simulink model "proxy"  (R2017b)
settings: Solver=ode3  StartTime=0.0  StopTime=inf  FixedStep=0.01  RelTol=1e-3  EnableMultiTasking=on
model workspace (MAT data in the model file):
  SL_ROS_VariableLengthArrays_MaxSizes : struct (value not decoded)
values from neighbouring files (symbols this model uses):
  filt = c2d(filt,sampleTime)    [Connect.m]
libraries: robotlib x8, simulink x6, simulink_extras x3, dspnetwork x3, etargetslib x2, xpcutilitieslib x1
(part 3 of 4)

== matlab function proxy/Generate SchunkCommands /Middle Finger/Jacobian2 ==
  data: pose input; sensor input; measurements input; JTcomp output single; q_next output; q_pr input; J22_old input; J22_ol output
function [JTcomp, q_next, J22_ol] = fcn( pose, sensor, measurements, q_pr, J22_old)
%#codegen
% JTcomp_T = zeros(1,2);
%JTcomp = zeros(1,2);

lx = sensor(1);
qB = sensor(2);

qo1 =pose(1);
qo2 =pose(2);
qK = pose(3);
qD = pose(4);
qG = pose(5);
qN = pose(6);
c1 = pose(7);
c2 = pose(8);

%POSE ESTIMATION VALUE
LIIp = measurements(2);
LJJp = LIIp;
LLM = measurements(1);

%LIIp= measurements(1);
%LJJp = measurements(2);
%LLM = measurements(3);
%offset = measurements(4);
%xL = measurements(5);


% LIIp = 7;
% LJJp = LIIp;
% LLM = 50;
% offset = 3;
xL = 10;

f1 = LLM;
f5 = xL;
LBH = 37; 
LKB = 35;
LKH = LKB + LBH;
LCI = 16;
LGH =  86;
LHG =  LGH;
LDE = 40;
LAB =  18;   
LEF =  27;
LGF =  46;
LCD =  9;
LBC =  43;
oy  = 134.8;
ox  = 15; 
LEJ =  39;
off_fing = LIIp;  
lact = 117.77;
% LKN =  135.6320;
LNO = lact;
LDF = LDE + LEF;
LBD = LBC + LCD;


stepsize = 0.01;

%%NEWEST (Jacobian_StiffnessRenderingOptimization_Sim.mdl)
q_dif = (sensor - q_pr) / stepsize;
q_dif1 = q_dif(1);
q_dif2 = q_dif(2);


J11 = -(cos(qo1)*(LKB*cos(qK)+LBC*cos(qB-qK)-LCI*sin(qB-qK))-sin(qo1)*(LKB*sin(qK)-LBC*sin(qB-qK)-LCI*cos(qB-qK)))*((LDE+LEF)*sin(qo2)*cos(qB-qD-qG)*(LKB*sin(qK)-LBC*sin(qB-qK)-LCI*cos(qB-qK))+(LDE+LEF)*sin(qN)^2*cos(qB-qD-qG)*(cos(qo1)*sin(qo1+qo2)*(LKB*sin(qK)-LBC*sin(qB-qK))-LCI*cos(qo1)*sin(qo1+qo2)*cos(qB-qK)-sin(qo2)*(LKB*sin(qK)-LBC*sin(qB-qK)-LCI*cos(qB-qK))-sin(qo1)*cos(qo1+qo2)*(LKB*sin(qK)-LBC*sin(qB-qK)-LCI*cos(qB-qK)))-cos(qo1)*((LDE+LEF)*cos(qB-qD-qG)*(cos(qo1+qo2)*(LCD*cos(qB-qK)+LCI*sin(qB-qK)+LDE*cos(qB-qD-qK)-LEJ*sin(qB-qD-qK))-sin(qo1+qo2)*(LCI*cos(qB-qK)-LCD*sin(qB-qK)-LDE*sin(qB-qD-qK)-LEJ*cos(qB-qD-qK)))+(sin(qo1+qo2)*(LDE*sin(qB-qD-qK)+LEJ*cos(qB-qD-qK))+cos(qo1+qo2)*(LDE*cos(qB-qD-qK)-LEJ*sin(qB-qD-qK)))*(cos(qG-qK)*(LBH*cos(qK)+LHG*sin(qK)-LBC*cos(qB-qK)-LCD*cos(qB-qK)-LDE*cos(qB-qD-qK)-LEF*cos(qB-qD-qK))+sin(qG-qK)*(LHG*cos(qK)-LBH*sin(qK)-LBC*sin(qB-qK)-LCD*sin(qB-qK)-LDE*sin(qB-qD-qK)-LEF*sin(qB-qD-qK)))))/(cos(qN)*(LKB*sin(qK)+LAB*sin(qB-qK)-tan(qN)*(LKB*cos(qK)-LAB*cos(qB-qK)))*((LDE+LEF)*sin(qo1)*sin(qo2)*cos(qB-qD-qG)*(LIIp*cos(qo1)-c1*sin(qo1))*(LKB*sin(qK)-LBC*sin(qB-qK)-LCI*cos(qB-qK))-cos(qo1)*((LIIp*sin(qo1)+c1*cos(qo1))*((LDE+LEF)*sin(qo2)*cos(qB-qD-qG)*(LKB*sin(qK)-LBC*sin(qB-qK)-LCI*cos(qB-qK))-cos(qo1)*((LDE+LEF)*cos(qB-qD-qG)*(cos(qo1+qo2)*(LCD*cos(qB-qK)+LCI*sin(qB-qK)+LDE*cos(qB-qD-qK)-LEJ*sin(qB-qD-qK))-sin(qo1+qo2)*(LCI*cos(qB-qK)-LCD*sin(qB-qK)-LDE*sin(qB-qD-qK)-LEJ*cos(qB-qD-qK)))+(sin(qo1+qo2)*(LDE*sin(qB-qD-qK)+LEJ*cos(qB-qD-qK))+cos(qo1+qo2)*(LDE*cos(qB-qD-qK)-LEJ*sin(qB-qD-qK)))*(cos(qG-qK)*(LBH*cos(qK)+LHG*sin(qK)-LBC*cos(qB-qK)-LCD*cos(qB-qK)-LDE*cos(qB-qD-qK)-LEF*cos(qB-qD-qK))+sin(qG-qK)*(LHG*cos(qK)-LBH*sin(qK)-LBC*sin(qB-qK)-LCD*sin(qB-qK)-LDE*sin(qB-qD-qK)-LEF*sin(qB-qD-qK)))))-sin(qo1)*(LIIp*cos(qo1)-c1*sin(qo1))*((LDE+LEF)*sin(qo1+qo2)*cos(qB-qD-qG)*(LCI*cos(qB-qK)-LCD*sin(qB-qK)-LDE*sin(qB-qD-qK)-LEJ*cos(qB-qD-qK))-sin(qo1+qo2)*(LDE*sin(qB-qD-qK)+LEJ*cos(qB-qD-qK))*(cos(qG-qK)*(LBH*cos(qK)+LHG*sin(qK)-LBC*cos(qB-qK)-LCD*cos(qB-qK)-LDE*cos(qB-qD-qK)-LEF*cos(qB-qD-qK))+sin(qG-qK)*(LHG*cos(qK)-LBH*sin(qK)-LBC*sin(qB-qK)-LCD*sin(qB-qK)-LDE*sin(qB-qD-qK)-LEF*sin(qB-qD-qK)))-cos(qo1+qo2)*((LDE+LEF)*cos(qG-qK)*cos(qB-qD-qK)*(LCD*cos(qB-qK)+LCI*sin(qB-qK)+LDE*cos(qB-qD-qK)-LEJ*sin(qB-qD-qK))+cos(qG-qK)*(LDE*cos(qB-qD-qK)-LEJ*sin(qB-qD-qK))*(LBH*cos(qK)+LHG*sin(qK)-LBC*cos(qB-qK)-LCD*cos(qB-qK)-LDE*cos(qB-qD-qK)-LEF*cos(qB-qD-qK))+sin(qG-qK)*((LDE+LEF)*sin(qB-qD-qK)*(LCD*cos(qB-qK)+LCI*sin(qB-qK)+LDE*cos(qB-qD-qK)-LEJ*sin(qB-qD-qK))+(LDE*cos(qB-qD-qK)-LEJ*sin(qB-qD-qK))*(LHG*cos(qK)-LBH*sin(qK)-LBC*sin(qB-qK)-LCD*sin(qB-qK)-LDE*sin(qB-qD-qK)-LEF*sin(qB-qD-qK))))))));
J12 = cos(qo1)*((LDE+LEF)*sin(qo1+qo2)*cos(qB-qD-qG)*(LCI*cos(qB-qK)-LCD*sin(qB-qK)-LDE*sin(qB-qD-qK)-LEJ*cos(qB-qD-qK))*(cos(qo1)*(LKB*cos(qK)+LBC*cos(qB-qK)-LCI*sin(qB-qK))-sin(qo1)*(LKB*sin(qK)-LBC*sin(qB-qK)-LCI*cos(qB-qK)))+sin(qG-qK)*(LBC*sin(qB-qK)+LCD*sin(qB-qK)+LDE*sin(qB-qD-qK)+LEF*sin(qB-qD-qK))*(sin(qo1+qo2)*(LDE*sin(qB-qD-qK)+LEJ*cos(qB-qD-qK))+cos(qo1+qo2)*(LDE*cos(qB-qD-qK)-LEJ*sin(qB-qD-qK)))*(cos(qo1)*(LKB*cos(qK)+LBC*cos(qB-qK)-LCI*sin(qB-qK))-sin(qo1)*(LKB*sin(qK)-LBC*sin(qB-qK)-LCI*cos(qB-qK)))+cos(qG-qK)*(LBC*cos(qB-qK)+LCD*cos(qB-qK)+LDE*cos(qB-qD-qK)+LEF*cos(qB-qD-qK))*(sin(qo1+qo2)*(LDE*sin(qB-qD-qK)+LEJ*cos(qB-qD-qK))+cos(qo1+qo2)*(LDE*cos(qB-qD-qK)-LEJ*sin(qB-qD-qK)))*(cos(qo1)*(LKB*cos(qK)+LBC*cos(qB-qK)-LCI*sin(qB-qK))-sin(qo1)*(LKB*sin(qK)-LBC*sin(qB-qK)-LCI*cos(qB-qK)))-(LDE+LEF)*cos(qo1+qo2)*cos(qB-qD-qG)*(LCD*cos(qB-qK)+LCI*sin(qB-qK)+LDE*cos(qB-qD-qK)-LEJ*sin(qB-qD-qK))*(cos(qo1)*(LKB*cos(qK)+LBC*cos(qB-qK)-LCI*sin(qB-qK))-sin(qo1)*(LKB*sin(qK)-LBC*sin(qB-qK)-LCI*cos(qB-qK)))-(LBC*cos(qB-qK)-LCI*sin(qB-qK))*((LDE+LEF)*sin(qo2)*cos(qB-qD-qG)*(LKB*sin(qK)-LBC*sin(qB-qK)-LCI*cos(qB-qK))-cos(qo1)*((LDE+LEF)*cos(qB-qD-qG)*(cos(qo1+qo2)*(LCD*cos(qB-qK)+LCI*sin(qB-qK)+LDE*cos(qB-qD-qK)-LEJ*sin(qB-qD-qK))-sin(qo1+qo2)*(LCI*cos(qB-qK)-LCD*sin(qB-qK)-LDE*sin(qB-qD-qK)-LEJ*cos(qB-qD-qK)))+(sin(qo1+qo2)*(LDE*sin(qB-qD-qK)+LEJ*cos(qB-qD-qK))+cos(qo1+qo2)*(LDE*cos(qB-qD-qK)-LEJ*sin(qB-qD-qK)))*(cos(qG-qK)*(LBH*cos(qK)+LHG*sin(qK)-LBC*cos(qB-qK)-LCD*cos(qB-qK)-LDE*cos(qB-qD-qK)-LEF*cos(qB-qD-qK))+sin(qG-qK)*(LHG*cos(qK)-LBH*sin(qK)-LBC*sin(qB-qK)-LCD*sin(qB-qK)-LDE*sin(qB-qD-qK)-LEF*sin(qB-qD-qK)))))-(LBC*sin(qB-qK)+LCI*cos(qB-qK))*((LDE+LEF)*sin(qo2)*cos(qB-qD-qG)*(LKB*cos(qK)+LBC*cos(qB-qK)-LCI*sin(qB-qK))+sin(qo1)*((LDE+LEF)*sin(qo1+qo2)*cos(qB-qD-qG)*(LCI*cos(qB-qK)-LCD*sin(qB-qK)-LDE*sin(qB-qD-qK)-LEJ*cos(qB-qD-qK))-sin(qo1+qo2)*(LDE*sin(qB-qD-qK)+LEJ*cos(qB-qD-qK))*(cos(qG-qK)*(LBH*cos(qK)+LHG*sin(qK)-LBC*cos(qB-qK)-LCD*cos(qB-qK)-LDE*cos(qB-qD-qK)-LEF*cos(qB-qD-qK))+sin(qG-qK)*(LHG*cos(qK)-LBH*sin(qK)-LBC*sin(qB-qK)-LCD*sin(qB-qK)-LDE*sin(qB-qD-qK)-LEF*sin(qB-qD-qK)))-cos(qo1+qo2)*((LDE+LEF)*cos(qG-qK)*cos(qB-qD-qK)*(LCD*cos(qB-qK)+LCI*sin(qB-qK)+LDE*cos(qB-qD-qK)-LEJ*sin(qB-qD-qK))+cos(qG-qK)*(LDE*cos(qB-qD-qK)-LEJ*sin(qB-qD-qK))*(LBH*cos(qK)+LHG*sin(qK)-LBC*cos(qB-qK)-LCD*cos(qB-qK)-LDE*cos(qB-qD-qK)-LEF*cos(qB-qD-qK))+sin(qG-qK)*((LDE+LEF)*sin(qB-qD-qK)*(LCD*cos(qB-qK)+LCI*sin(qB-qK)+LDE*cos(qB-qD-qK)-LEJ*sin(qB-qD-qK))+(LDE*cos(qB-qD-qK)-LEJ*sin(qB-qD-qK))*(LHG*cos(qK)-LBH*sin(qK)-LBC*sin(qB-qK)-LCD*sin(qB-qK)-LDE*sin(qB-qD-qK)-LEF*sin(qB-qD-qK)))))))/((LDE+LEF)*sin(qo1)*sin(qo2)*cos(qB-qD-qG)*(LIIp*cos(qo1)-c1*sin(qo1))*(LKB*sin(qK)-LBC*sin(qB-qK)-LCI*cos(qB-qK))-cos(qo1)*((LIIp*sin(qo1)+c1*cos(qo1))*((LDE+LEF)*sin(qo2)*cos(qB-qD-qG)*(LKB*sin(qK)-LBC*sin(qB-qK)-LCI*cos(qB-qK))-cos(qo1)*((LDE+LEF)*cos(qB-qD-qG)*(cos(qo1+qo2)*(LCD*cos(qB-qK)+LCI*sin(qB-qK)+LDE*cos(qB-qD-qK)-LEJ*sin(qB-qD-qK))-sin(qo1+qo2)*(LCI*cos(qB-qK)-LCD*sin(qB-qK)-LDE*sin(qB-qD-qK)-LEJ*cos(qB-qD-qK)))+(sin(qo1+qo2)*(LDE*sin(qB-qD-qK)+LEJ*cos(qB-qD-qK))+cos(qo1+qo2)*(LDE*cos(qB-qD-qK)-LEJ*sin(qB-qD-qK)))*(cos(qG-qK)*(LBH*cos(qK)+LHG*sin(qK)-LBC*cos(qB-qK)-LCD*cos(qB-qK)-LDE*cos(qB-qD-qK)-LEF*cos(qB-qD-qK))+sin(qG-qK)*(LHG*cos(qK)-LBH*sin(qK)-LBC*sin(qB-qK)-LCD*sin(qB-qK)-LDE*sin(qB-qD-qK)-LEF*sin(qB-qD-qK)))))-sin(qo1)*(LIIp*cos(qo1)-c1*sin(qo1))*((LDE+LEF)*sin(qo1+qo2)*cos(qB-qD-qG)*(LCI*cos(qB-qK)-LCD*sin(qB-qK)-LDE*sin(qB-qD-qK)-LEJ*cos(qB-qD-qK))-sin(qo1+qo2)*(LDE*sin(qB-qD-qK)+LEJ*cos(qB-qD-qK))*(cos(qG-qK)*(LBH*cos(qK)+LHG*sin(qK)-LBC*cos(qB-qK)-LCD*cos(qB-qK)-LDE*cos(qB-qD-qK)-LEF*cos(qB-qD-qK))+sin(qG-qK)*(LHG*cos(qK)-LBH*sin(qK)-LBC*sin(qB-qK)-LCD*sin(qB-qK)-LDE*sin(qB-qD-qK)-LEF*sin(qB-qD-qK)))-cos(qo1+qo2)*((LDE+LEF)*cos(qG-qK)*cos(qB-qD-qK)*(LCD*cos(qB-qK)+LCI*sin(qB-qK)+LDE*cos(qB-qD-qK)-LEJ*sin(qB-qD-qK))+cos(qG-qK)*(LDE*cos(qB-qD-qK)-LEJ*sin(qB-qD-qK))*(LBH*cos(qK)+LHG*sin(qK)-LBC*cos(qB-qK)-LCD*cos(qB-qK)-LDE*cos(qB-qD-qK)-LEF*cos(qB-qD-qK))+sin(qG-qK)*((LDE+LEF)*sin(qB-qD-qK)*(LCD*cos(qB-qK)+LCI*sin(qB-qK)+LDE*cos(qB-qD-qK)-LEJ*sin(qB-qD-qK))+(LDE*cos(qB-qD-qK)-LEJ*sin(qB-qD-qK))*(LHG*cos(qK)-LBH*sin(qK)-LBC*sin(qB-qK)-LCD*sin(qB-qK)-LDE*sin(qB-qD-qK)-LEF*sin(qB-qD-qK))))))) - (cos(qo1)*(LKB*cos(qK)+LBC*cos(qB-qK)-LCI*sin(qB-qK))-sin(qo1)*(LKB*sin(qK)-LBC*sin(qB-qK)-LCI*cos(qB-qK)))*((LDE+LEF)*cos(qo1)*sin(qo1+qo2)*cos(qB-qD-qG)*(LKB*sin(qK)+LAB*sin(qB-qK)-tan(qN)*(LKB*cos(qK)-LAB*cos(qB-qK)))*(LCI*cos(qB-qK)-LCD*sin(qB-qK)-LDE*sin(qB-qD-qK)-LEJ*cos(qB-qD-qK))+cos(qo1)*sin(qG-qK)*(LKB*sin(qK)+LAB*sin(qB-qK)-tan(qN)*(LKB*cos(qK)-LAB*cos(qB-qK)))*(LBC*sin(qB-qK)+LCD*sin(qB-qK)+LDE*sin(qB-qD-qK)+LEF*sin(qB-qD-qK))*(sin(qo1+qo2)*(LDE*sin(qB-qD-qK)+LEJ*cos(qB-qD-qK))+cos(qo1+qo2)*(LDE*cos(qB-qD-qK)-LEJ*sin(qB-qD-qK)))+cos(qo1)*cos(qG-qK)*(LKB*sin(qK)+LAB*sin(qB-qK)-tan(qN)*(LKB*cos(qK)-LAB*cos(qB-qK)))*(LBC*cos(qB-qK)+LCD*cos(qB-qK)+LDE*cos(qB-qD-qK)+LEF*cos(qB-qD-qK))*(sin(qo1+qo2)*(LDE*sin(qB-qD-qK)+LEJ*cos(qB-qD-qK))+cos(qo1+qo2)*(LDE*cos(qB-qD-qK)-LEJ*sin(qB-qD-qK)))-(LDE+LEF)*sin(qo2)*cos(qB-qD-qG)*(LBC*sin(qB-qK)+LCI*cos(qB-qK))*(LKB*sin(qK)+LAB*sin(qB-qK)-tan(qN)*(LKB*cos(qK)-LAB*cos(qB-qK)))-(LDE+LEF)*cos(qo1)*cos(qo1+qo2)*cos(qB-qD-qG)*(LKB*sin(qK)+LAB*sin(qB-qK)-tan(qN)*(LKB*cos(qK)-LAB*cos(qB-qK)))*(LCD*cos(qB-qK)+LCI*sin(qB-qK)+LDE*cos(qB-qD-qK)-LEJ*sin(qB-qD-qK))-LAB*sin(qB-qK)*((LDE+LEF)*sin(qo2)*cos(qB-qD-qG)*(LKB*sin(qK)-LBC*sin(qB-qK)-LCI*cos(qB-qK))-cos(qo1)*((LDE+LEF)*cos(qB-qD-qG)*(cos(qo1+qo2)*(LCD*cos(qB-qK)+LCI*sin(qB-qK)+LDE*cos(qB-qD-qK)-LEJ*sin(qB-qD-qK))-sin(qo1+qo2)*(LCI*cos(qB-qK)-LCD*sin(qB-qK)-LDE*sin(qB-qD-qK)-LEJ*cos(qB-qD-qK)))+(sin(qo1+qo2)*(LDE*sin(qB-qD-qK)+LEJ*cos(qB-qD-qK))+cos(qo1+qo2)*(LDE*cos(qB-qD-qK)-LEJ*sin(qB-qD-qK)))*(cos(qG-qK)*(LBH*cos(qK)+LHG*sin(qK)-LBC*cos(qB-qK)-LCD*cos(qB-qK)-LDE*cos(qB-qD-qK)-LEF*cos(qB-qD-qK))+sin(qG-qK)*(LHG*cos(qK)-LBH*sin(qK)-LBC*sin(qB-qK)-LCD*sin(qB-qK)-LDE*sin(qB-qD-qK)-LEF*sin(qB-qD-qK)))))-LAB*tan(qN)*cos(qB-qK)*((LDE+LEF)*cos(qo1)*sin(qo1+qo2)*cos(qB-qD-qG)*(LKB*sin(qK)-LBC*sin(qB-qK)-LCD*sin(qB-qK)-LDE*sin(qB-qD-qK)-LEJ*cos(qB-qD-qK))-(LDE+LEF)*sin(qo1)*cos(qo1+qo2)*cos(qB-qD-qG)*(LKB*sin(qK)-LBC*sin(qB-qK)-LCI*cos(qB-qK))-cos(qo1)*sin(qo1+qo2)*(LDE*sin(qB-qD-qK)+LEJ*cos(qB-qD-qK))*(cos(qG-qK)*(LBH*cos(qK)+LHG*sin(qK)-LBC*cos(qB-qK)-LCD*cos(qB-qK)-LDE*cos(qB-qD-qK)-LEF*cos(qB-qD-qK))+sin(qG-qK)*(LHG*cos(qK)-LBH*sin(qK)-LBC*sin(qB-qK)-LCD*sin(qB-qK)-LDE*sin(qB-qD-qK)-LEF*sin(qB-qD-qK)))-cos(qo1)*cos(qo1+qo2)*((LDE+LEF)*cos(qG-qK)*cos(qB-qD-qK)*(LCD*cos(qB-qK)+LCI*sin(qB-qK)+LDE*cos(qB-qD-qK)-LEJ*sin(qB-qD-qK))+cos(qG-qK)*(LDE*cos(qB-qD-qK)-LEJ*sin(qB-qD-qK))*(LBH*cos(qK)+LHG*sin(qK)-LBC*cos(qB-qK)-LCD*cos(qB-qK)-LDE*cos(qB-qD-qK)-LEF*cos(qB-qD-qK))+sin(qG-qK)*((LDE+LEF)*sin(qB-qD-qK)*(LCD*cos(qB-qK)+LCI*sin(qB-qK)+LDE*cos(qB-qD-qK)-LEJ*sin(qB-qD-qK))+(LDE*cos(qB-qD-qK)-LEJ*sin(qB-qD-qK))*(LHG*cos(qK)-LBH*sin(qK)-LBC*sin(qB-qK)-LCD*sin(qB-qK)-LDE*sin(qB-qD-qK)-LEF*sin(qB-qD-qK))))))/((LKB*sin(qK)+LAB*sin(qB-qK)-tan(qN)*(LKB*cos(qK)-LAB*cos(qB-qK)))*((LDE+LEF)*sin(qo1)*sin(qo2)*cos(qB-qD-qG)*(LIIp*cos(qo1)-c1*sin(qo1))*(LKB*sin(qK)-LBC*sin(qB-qK)-LCI*cos(qB-qK))-cos(qo1)*((LIIp*sin(qo1)+c1*cos(qo1))*((LDE+LEF)*sin(qo2)*cos(qB-qD-qG)*(LKB*sin(qK)-LBC*sin(qB-qK)-LCI*cos(qB-qK))-cos(qo1)*((LDE+LEF)*cos(qB-qD-qG)*(cos(qo1+qo2)*(LCD*cos(qB-qK)+LCI*sin(qB-qK)+LDE*cos(qB-qD-qK)-LEJ*sin(qB-qD-qK))-sin(qo1+qo2)*(LCI*cos(qB-qK)-LCD*sin(qB-qK)-LDE*sin(qB-qD-qK)-LEJ*cos(qB-qD-qK)))+(sin(qo1+qo2)*(LDE*sin(qB-qD-qK)+LEJ*cos(qB-qD-qK))+cos(qo1+qo2)*(LDE*cos(qB-qD-qK)-LEJ*sin(qB-qD-qK)))*(cos(qG-qK)*(LBH*cos(qK)+LHG*sin(qK)-LBC*cos(qB-qK)-LCD*cos(qB-qK)-LDE*cos(qB-qD-qK)-LEF*cos(qB-qD-qK))+sin(qG-qK)*(LHG*cos(qK)-LBH*sin(qK)-LBC*sin(qB-qK)-LCD*sin(qB-qK)-LDE*sin(qB-qD-qK)-LEF*sin(qB-qD-qK)))))-sin(qo1)*(LIIp*cos(qo1)-c1*sin(qo1))*((LDE+LEF)*sin(qo1+qo2)*cos(qB-qD-qG)*(LCI*cos(qB-qK)-LCD*sin(qB-qK)-LDE*sin(qB-qD-qK)-LEJ*cos(qB-qD-qK))-sin(qo1+qo2)*(LDE*sin(qB-qD-qK)+LEJ*cos(qB-qD-qK))*(cos(qG-qK)*(LBH*cos(qK)+LHG*sin(qK)-LBC*cos(qB-qK)-LCD*cos(qB-qK)-LDE*cos(qB-qD-qK)-LEF*cos(qB-qD-qK))+sin(qG-qK)*(LHG*cos(qK)-LBH*sin(qK)-LBC*sin(qB-qK)-LCD*sin(qB-qK)-LDE*sin(qB-qD-qK)-LEF*sin(qB-qD-qK)))-cos(qo1+qo2)*((LDE+LEF)*cos(qG-qK)*cos(qB-qD-qK)*(LCD*cos(qB-qK)+LCI*sin(qB-qK)+LDE*cos(qB-qD-qK)-LEJ*sin(qB-qD-qK))+cos(qG-qK)*(LDE*cos(qB-qD-qK)-LEJ*sin(qB-qD-qK))*(LBH*cos(qK)+LHG*sin(qK)-LBC*cos(qB-qK)-LCD*cos(qB-qK)-LDE*cos(qB-qD-qK)-LEF*cos(qB-qD-qK))+sin(qG-qK)*((LDE+LEF)*sin(qB-qD-qK)*(LCD*cos(qB-qK)+LCI*sin(qB-qK)+LDE*cos(qB-qD-qK)-LEJ*sin(qB-qD-qK))+(LDE*cos(qB-qD-qK)-LEJ*sin(qB-qD-qK))*(LHG*cos(qK)-LBH*sin(qK)-LBC*sin(qB-qK)-LCD*sin(qB-qK)-LDE*sin(qB-qD-qK)-LEF*sin(qB-qD-qK))))))));
J21 = -(((LDE+LEF)*sin(qo2)*cos(qB-qD-qG)*(LKB*sin(qK)-LBC*sin(qB-qK)-LCI*cos(qB-qK))-cos(qo1)*((LDE+LEF)*cos(qB-qD-qG)*(cos(qo1+qo2)*(LCD*cos(qB-qK)+LCI*sin(qB-qK)+LDE*cos(qB-qD-qK)-LEJ*sin(qB-qD-qK))-sin(qo1+qo2)*(LCI*cos(qB-qK)-LCD*sin(qB-qK)-LDE*sin(qB-qD-qK)-LEJ*cos(qB-qD-qK)))+(sin(qo1+qo2)*(LDE*sin(qB-qD-qK)+LEJ*cos(qB-qD-qK))+cos(qo1+qo2)*(LDE*cos(qB-qD-qK)-LEJ*sin(qB-qD-qK)))*(cos(qG-qK)*(LBH*cos(qK)+LHG*sin(qK)-LBC*cos(qB-qK)-LCD*cos(qB-qK)-LDE*cos(qB-qD-qK)-LEF*cos(qB-qD-qK))+sin(qG-qK)*(LHG*cos(qK)-LBH*sin(qK)-LBC*sin(qB-qK)-LCD*sin(qB-qK)-LDE*sin(qB-qD-qK)-LEF*sin(qB-qD-qK)))))^2*(cos(qN)+sin(qN)^2*((LDE+LEF)*cos(qo1)*sin(qo1+qo2)*cos(qB-qD-qG)*(LKB*sin(qK)-LBC*sin(qB-qK)-LCD*sin(qB-qK)-LDE*sin(qB-qD-qK)-LEJ*cos(qB-qD-qK))-(LDE+LEF)*sin(qo1)*cos(qo1+qo2)*cos(qB-qD-qG)*(LKB*sin(qK)-LBC*sin(qB-qK)-LCI*cos(qB-qK))-cos(qo1)*sin(qo1+qo2)*(LDE*sin(qB-qD-qK)+LEJ*cos(qB-qD-qK))*(cos(qG-qK)*(LBH*cos(qK)+LHG*sin(qK)-LBC*cos(qB-qK)-LCD*cos(qB-qK)-LDE*cos(qB-qD-qK)-LEF*cos(qB-qD-qK))+sin(qG-qK)*(LHG*cos(qK)-LBH*sin(qK)-LBC*sin(qB-qK)-LCD*sin(qB-qK)-LDE*sin(qB-qD-qK)-LEF*sin(qB-qD-qK)))-cos(qo1)*cos(qo1+qo2)*((LDE+LEF)*cos(qG-qK)*cos(qB-qD-qK)*(LCD*cos(qB-qK)+LCI*sin(qB-qK)+LDE*cos(qB-qD-qK)-LEJ*sin(qB-qD-qK))+cos(qG-qK)*(LDE*cos(qB-qD-qK)-LEJ*sin(qB-qD-qK))*(LBH*cos(qK)+LHG*sin(qK)-LBC*cos(qB-qK)-LCD*cos(qB-qK)-LDE*cos(qB-qD-qK)-LEF*cos(qB-qD-qK))+sin(qG-qK)*((LDE+LEF)*sin(qB-qD-qK)*(LCD*cos(qB-qK)+LCI*sin(qB-qK)+LDE*cos(qB-qD-qK)-LEJ*sin(qB-qD-qK))+(LDE*cos(qB-qD-qK)-LEJ*sin(qB-qD-qK))*(LHG*cos(qK)-LBH*sin(qK)-LBC*sin(qB-qK)-LCD*sin(qB-qK)-LDE*sin(qB-qD-qK)-LEF*sin(qB-qD-qK)))))/(cos(qN)*((LDE+LEF)*sin(qo2)*cos(qB-qD-qG)*(LKB*sin(qK)-LBC*sin(qB-qK)-LCI*cos(qB-qK))-cos(qo1)*((LDE+LEF)*cos(qB-qD-qG)*(cos(qo1+qo2)*(LCD*cos(qB-qK)+LCI*sin(qB-qK)+LDE*cos(qB-qD-qK)-LEJ*sin(qB-qD-qK))-sin(qo1+qo2)*(LCI*cos(qB-qK)-LCD*sin(qB-qK)-LDE*sin(qB-qD-qK)-LEJ*cos(qB-qD-qK)))+(sin(qo1+qo2)*(LDE*sin(qB-qD-qK)+LEJ*cos(qB-qD-qK))+cos(qo1+qo2)*(LDE*cos(qB-qD-qK)-LEJ*sin(qB-qD-qK)))*(cos(qG-qK)*(LBH*cos(qK)+LHG*sin(qK)-LBC*cos(qB-qK)-LCD*cos(qB-qK)-LDE*cos(qB-qD-qK)-LEF*cos(qB-qD-qK))+sin(qG-qK)*(LHG*cos(qK)-LBH*sin(qK)-LBC*sin(qB-qK)-LCD*sin(qB-qK)-LDE*sin(qB-qD-qK)-LEF*sin(qB-qD-qK)))))))*(LIIp*sin(qo1)+c1*cos(qo1)+((LDE+LEF)*c2*cos(qB-qD-qG)*(cos(qo1)*(LKB*cos(qK)+LBC*cos(qB-qK)-LCI*sin(qB-qK))-sin(qo1)*(LKB*sin(qK)-LBC*sin(qB-qK)-LCI*cos(qB-qK)))+(LDE+LEF)*sin(qo1+qo2)*cos(qB-qD-qG)*(LIIp*cos(qo1)+sin(qo1)*(LLM-c1))*(cos(qo1)*(LKB*cos(qK)+LBC*cos(qB-qK)-LCI*sin(qB-qK))-sin(qo1)*(LKB*sin(qK)-LBC*sin(qB-qK)-LCI*cos(qB-qK)))-(LDE+LEF)*cos(qo1+qo2)*cos(qB-qD-qG)*(LIIp*sin(qo1)-cos(qo1)*(LLM-c1))*(cos(qo1)*(LKB*cos(qK)+LBC*cos(qB-qK)-LCI*sin(qB-qK))-sin(qo1)*(LKB*sin(qK)-LBC*sin(qB-qK)-LCI*cos(qB-qK)))-(LIIp*cos(qo1)-c1*sin(qo1))*((LDE+LEF)*sin(qo2)*cos(qB-qD-qG)*(LKB*cos(qK)+LBC*cos(qB-qK)-LCI*sin(qB-qK))+sin(qo1)*((LDE+LEF)*sin(qo1+qo2)*cos(qB-qD-qG)*(LCI*cos(qB-qK)-LCD*sin(qB-qK)-LDE*sin(qB-qD-qK)-LEJ*cos(qB-qD-qK))-sin(qo1+qo2)*(LDE*sin(qB-qD-qK)+LEJ*cos(qB-qD-qK))*(cos(qG-qK)*(LBH*cos(qK)+LHG*sin(qK)-LBC*cos(qB-qK)-LCD*cos(qB-qK)-LDE*cos(qB-qD-qK)-LEF*cos(qB-qD-qK))+sin(qG-qK)*(LHG*cos(qK)-LBH*sin(qK)-LBC*sin(qB-qK)-LCD*sin(qB-qK)-LDE*sin(qB-qD-qK)-LEF*sin(qB-qD-qK)))-cos(qo1+qo2)*((LDE+LEF)*cos(qG-qK)*cos(qB-qD-qK)*(LCD*cos(qB-qK)+LCI*sin(qB-qK)+LDE*cos(qB-qD-qK)-LEJ*sin(qB-qD-qK))+cos(qG-qK)*(LDE*cos(qB-qD-qK)-LEJ*sin(qB-qD-qK))*(LBH*cos(qK)+LHG*sin(qK)-LBC*cos(qB-qK)-LCD*cos(qB-qK)-LDE*cos(qB-qD-qK)-LEF*cos(qB-qD-qK))+sin(qG-qK)*((LDE+LEF)*sin(qB-qD-qK)*(LCD*cos(qB-qK)+LCI*sin(qB-qK)+LDE*cos(qB-qD-qK)-LEJ*sin(qB-qD-qK))+(LDE*cos(qB-qD-qK)-LEJ*sin(qB-qD-qK))*(LHG*cos(qK)-LBH*sin(qK)-LBC*sin(qB-qK)-LCD*sin(qB-qK)-LDE*sin(qB-qD-qK)-LEF*sin(qB-qD-qK)))))))/((LDE+LEF)*sin(qo2)*cos(qB-qD-qG)*(LKB*sin(qK)-LBC*sin(qB-qK)-LCI*cos(qB-qK))-cos(qo1)*((LDE+LEF)*cos(qB-qD-qG)*(cos(qo1+qo2)*(LCD*cos(qB-qK)+LCI*sin(qB-qK)+LDE*cos(qB-qD-qK)-LEJ*sin(qB-qD-qK))-sin(qo1+qo2)*(LCI*cos(qB-qK)-LCD*sin(qB-qK)-LDE*sin(qB-qD-qK)-LEJ*cos(qB-qD-qK)))+(sin(qo1+qo2)*(LDE*sin(qB-qD-qK)+LEJ*cos(qB-qD-qK))+cos(qo1+qo2)*(LDE*cos(qB-qD-qK)-LEJ*sin(qB-qD-qK)))*(cos(qG-qK)*(LBH*cos(qK)+LHG*sin(qK)-LBC*cos(qB-qK)-LCD*cos(qB-qK)-LDE*cos(qB-qD-qK)-LEF*cos(qB-qD-qK))+sin(qG-qK)*(LHG*cos(qK)-LBH*sin(qK)-LBC*sin(qB-qK)-LCD*sin(qB-qK)-LDE*sin(qB-qD-qK)-LEF*sin(qB-qD-qK))))))/((LDE+LEF)*c2*cos(qB-qD-qG)*(LKB*sin(qK)+LAB*sin(qB-qK)-tan(qN)*(LKB*cos(qK)-LAB*cos(qB-qK)))*((LDE+LEF)*sin(qo1)*sin(qo2)*cos(qB-qD-qG)*(LIIp*cos(qo1)-c1*sin(qo1))*(LKB*sin(qK)-LBC*sin(qB-qK)-LCI*cos(qB-qK))-cos(qo1)*((LIIp*sin(qo1)+c1*cos(qo1))*((LDE+LEF)*sin(qo2)*cos(qB-qD-qG)*(LKB*sin(qK)-LBC*sin(qB-qK)-LCI*cos(qB-qK))-cos(qo1)*((LDE+LEF)*cos(qB-qD-qG)*(cos(qo1+qo2)*(LCD*cos(qB-qK)+LCI*sin(qB-qK)+LDE*cos(qB-qD-qK)-LEJ*sin(qB-qD-qK))-sin(qo1+qo2)*(LCI*cos(qB-qK)-LCD*sin(qB-qK)-LDE*sin(qB-qD-qK)-LEJ*cos(qB-qD-qK)))+(sin(qo1+qo2)*(LDE*sin(qB-qD-qK)+LEJ*cos(qB-qD-qK))+cos(qo1+qo2)*(LDE*cos(qB-qD-qK)-LEJ*sin(qB-qD-qK)))*(cos(qG-qK)*(LBH*cos(qK)+LHG*sin(qK)-LBC*cos(qB-qK)-LCD*cos(qB-qK)-LDE*cos(qB-qD-qK)-LEF*cos(qB-qD-qK))+sin(qG-qK)*(LHG*cos(qK)-LBH*sin(qK)-LBC*sin(qB-qK)-LCD*sin(qB-qK)-LDE*sin(qB-qD-qK)-LEF*sin(qB-qD-qK)))))-sin(qo1)*(LIIp*cos(qo1)-c1*sin(qo1))*((LDE+LEF)*sin(qo1+qo2)*cos(qB-qD-qG)*(LCI*cos(qB-qK)-LCD*sin(qB-qK)-LDE*sin(qB-qD-qK)-LEJ*cos(qB-qD-qK))-sin(qo1+qo2)*(LDE*sin(qB-qD-qK)+LEJ*cos(qB-qD-qK))*(cos(qG-qK)*(LBH*cos(qK)+LHG*sin(qK)-LBC*cos(qB-qK)-LCD*cos(qB-qK)-LDE*cos(qB-qD-qK)-LEF*cos(qB-qD-qK))+sin(qG-qK)*(LHG*cos(qK)-LBH*sin(qK)-LBC*sin(qB-qK)-LCD*sin(qB-qK)-LDE*sin(qB-qD-qK)-LEF*sin(qB-qD-qK)))-cos(qo1+qo2)*((LDE+LEF)*cos(qG-qK)*cos(qB-qD-qK)*(LCD*cos(qB-qK)+LCI*sin(qB-qK)+LDE*cos(qB-qD-qK)-LEJ*sin(qB-qD-qK))+cos(qG-qK)*(LDE*cos(qB-qD-qK)-LEJ*sin(qB-qD-qK))*(LBH*cos(qK)+LHG*sin(qK)-LBC*cos(qB-qK)-LCD*cos(qB-qK)-LDE*cos(qB-qD-qK)-LEF*cos(qB-qD-qK))+sin(qG-qK)*((LDE+LEF)*sin(qB-qD-qK)*(LCD*cos(qB-qK)+LCI*sin(qB-qK)+LDE*cos(qB-qD-qK)-LEJ*sin(qB-qD-qK))+(LDE*cos(qB-qD-qK)-LEJ*sin(qB-qD-qK))*(LHG*cos(qK)-LBH*sin(qK)-LBC*sin(qB-qK)-LCD*sin(qB-qK)-LDE*sin(qB-qD-qK)-LEF*sin(qB-qD-qK)))))))));
J22_c = (-(c2*cos(qo1)+cos(qo1)*sin(qo1+qo2)*(LIIp*cos(qo1)+sin(qo1)*(LLM-c1))-sin(qo2)*(LIIp*cos(qo1)-c1*sin(qo1))-cos(qo1)*cos(qo1+qo2)*(LIIp*sin(qo1)-cos(qo1)*(LLM-c1)))*((LDE+LEF)*sin(qo1+qo2)*cos(qB-qD-qG)*(LCI*cos(qB-qK)-LCD*sin(qB-qK)-LDE*sin(qB-qD-qK)-LEJ*cos(qB-qD-qK))*(cos(qo1)*(LKB*cos(qK)+LBC*cos(qB-qK)-LCI*sin(qB-qK))-sin(qo1)*(LKB*sin(qK)-LBC*sin(qB-qK)-LCI*cos(qB-qK)))+sin(qG-qK)*(LBC*sin(qB-qK)+LCD*sin(qB-qK)+LDE*sin(qB-qD-qK)+LEF*sin(qB-qD-qK))*(sin(qo1+qo2)*(LDE*sin(qB-qD-qK)+LEJ*cos(qB-qD-qK))+cos(qo1+qo2)*(LDE*cos(qB-qD-qK)-LEJ*sin(qB-qD-qK)))*(cos(qo1)*(LKB*cos(qK)+LBC*cos(qB-qK)-LCI*sin(qB-qK))-sin(qo1)*(LKB*sin(qK)-LBC*sin(qB-qK)-LCI*cos(qB-qK)))+cos(qG-qK)*(LBC*cos(qB-qK)+LCD*cos(qB-qK)+LDE*cos(qB-qD-qK)+LEF*cos(qB-qD-qK))*(sin(qo1+qo2)*(LDE*sin(qB-qD-qK)+LEJ*cos(qB-qD-qK))+cos(qo1+qo2)*(LDE*cos(qB-qD-qK)-LEJ*sin(qB-qD-qK)))*(cos(qo1)*(LKB*cos(qK)+LBC*cos(qB-qK)-LCI*sin(qB-qK))-sin(qo1)*(LKB*sin(qK)-LBC*sin(qB-qK)-LCI*cos(qB-qK)))-(LDE+LEF)*cos(qo1+qo2)*cos(qB-qD-qG)*(LCD*cos(qB-qK)+LCI*sin(qB-qK)+LDE*cos(qB-qD-qK)-LEJ*sin(qB-qD-qK))*(cos(qo1)*(LKB*cos(qK)+LBC*cos(qB-qK)-LCI*sin(qB-qK))-sin(qo1)*(LKB*sin(qK)-LBC*sin(qB-qK)-LCI*cos(qB-qK)))-(LBC*cos(qB-qK)-LCI*sin(qB-qK))*((LDE+LEF)*sin(qo2)*cos(qB-qD-qG)*(LKB*sin(qK)-LBC*sin(qB-qK)-LCI*cos(qB-qK))-cos(qo1)*((LDE+LEF)*cos(qB-qD-qG)*(cos(qo1+qo2)*(LCD*cos(qB-qK)+LCI*sin(qB-qK)+LDE*cos(qB-qD-qK)-LEJ*sin(qB-qD-qK))-sin(qo1+qo2)*(LCI*cos(qB-qK)-LCD*sin(qB-qK)-LDE*sin(qB-qD-qK)-LEJ*cos(qB-qD-qK)))+(sin(qo1+qo2)*(LDE*sin(qB-qD-qK)+LEJ*cos(qB-qD-qK))+cos(qo1+qo2)*(LDE*cos(qB-qD-qK)-LEJ*sin(qB-qD-qK)))*(cos(qG-qK)*(LBH*cos(qK)+LHG*sin(qK)-LBC*cos(qB-qK)-LCD*cos(qB-qK)-LDE*cos(qB-qD-qK)-LEF*cos(qB-qD-qK))+sin(qG-qK)*(LHG*cos(qK)-LBH*sin(qK)-LBC*sin(qB-qK)-LCD*sin(qB-qK)-LDE*sin(qB-qD-qK)-LEF*sin(qB-qD-qK)))))-(LBC*sin(qB-qK)+LCI*cos(qB-qK))*((LDE+LEF)*sin(qo2)*cos(qB-qD-qG)*(LKB*cos(qK)+LBC*cos(qB-qK)-LCI*sin(qB-qK))+sin(qo1)*((LDE+LEF)*sin(qo1+qo2)*cos(qB-qD-qG)*(LCI*cos(qB-qK)-LCD*sin(qB-qK)-LDE*sin(qB-qD-qK)-LEJ*cos(qB-qD-qK))-sin(qo1+qo2)*(LDE*sin(qB-qD-qK)+LEJ*cos(qB-qD-qK))*(cos(qG-qK)*(LBH*cos(qK)+LHG*sin(qK)-LBC*cos(qB-qK)-LCD*cos(qB-qK)-LDE*cos(qB-qD-qK)-LEF*cos(qB-qD-qK))+sin(qG-qK)*(LHG*cos(qK)-LBH*sin(qK)-LBC*sin(qB-qK)-LCD*sin(qB-qK)-LDE*sin(qB-qD-qK)-LEF*sin(qB-qD-qK)))-cos(qo1+qo2)*((LDE+LEF)*cos(qG-qK)*cos(qB-qD-qK)*(LCD*cos(qB-qK)+LCI*sin(qB-qK)+LDE*cos(qB-qD-qK)-LEJ*sin(qB-qD-qK))+cos(qG-qK)*(LDE*cos(qB-qD-qK)-LEJ*sin(qB-qD-qK))*(LBH*cos(qK)+LHG*sin(qK)-LBC*cos(qB-qK)-LCD*cos(qB-qK)-LDE*cos(qB-qD-qK)-LEF*cos(qB-qD-qK))+sin(qG-qK)*((LDE+LEF)*sin(qB-qD-qK)*(LCD*cos(qB-qK)+LCI*sin(qB-qK)+LDE*cos(qB-qD-qK)-LEJ*sin(qB-qD-qK))+(LDE*cos(qB-qD-qK)-LEJ*sin(qB-qD-qK))*(LHG*cos(qK)-LBH*sin(qK)-LBC*sin(qB-qK)-LCD*sin(qB-qK)-LDE*sin(qB-qD-qK)-LEF*sin(qB-qD-qK)))))))/(c2*((LDE+LEF)*sin(qo1)*sin(qo2)*cos(qB-qD-qG)*(LIIp*cos(qo1)-c1*sin(qo1))*(LKB*sin(qK)-LBC*sin(qB-qK)-LCI*cos(qB-qK))-cos(qo1)*((LIIp*sin(qo1)+c1*cos(qo1))*((LDE+LEF)*sin(qo2)*cos(qB-qD-qG)*(LKB*sin(qK)-LBC*sin(qB-qK)-LCI*cos(qB-qK))-cos(qo1)*((LDE+LEF)*cos(qB-qD-qG)*(cos(qo1+qo2)*(LCD*cos(qB-qK)+LCI*sin(qB-qK)+LDE*cos(qB-qD-qK)-LEJ*sin(qB-qD-qK))-sin(qo1+qo2)*(LCI*cos(qB-qK)-LCD*sin(qB-qK)-LDE*sin(qB-qD-qK)-LEJ*cos(qB-qD-qK)))+(sin(qo1+qo2)*(LDE*sin(qB-qD-qK)+LEJ*cos(qB-qD-qK))+cos(qo1+qo2)*(LDE*cos(qB-qD-qK)-LEJ*sin(qB-qD-qK)))*(cos(qG-qK)*(LBH*cos(qK)+LHG*sin(qK)-LBC*cos(qB-qK)-LCD*cos(qB-qK)-LDE*cos(qB-qD-qK)-LEF*cos(qB-qD-qK))+sin(qG-qK)*(LHG*cos(qK)-LBH*sin(qK)-LBC*sin(qB-qK)-LCD*sin(qB-qK)-LDE*sin(qB-qD-qK)-LEF*sin(qB-qD-qK)))))-sin(qo1)*(LIIp*cos(qo1)-c1*sin(qo1))*((LDE+LEF)*sin(qo1+qo2)*cos(qB-qD-qG)*(LCI*cos(qB-qK)-LCD*sin(qB-qK)-LDE*sin(qB-qD-qK)-LEJ*cos(qB-qD-qK))-sin(qo1+qo2)*(LDE*sin(qB-qD-qK)+LEJ*cos(qB-qD-qK))*(cos(qG-qK)*(LBH*cos(qK)+LHG*sin(qK)-LBC*cos(qB-qK)-LCD*cos(qB-qK)-LDE*cos(qB-qD-qK)-LEF*cos(qB-qD-qK))+sin(qG-qK)*(LHG*cos(qK)-LBH*sin(qK)-LBC*sin(qB-qK)-LCD*sin(qB-qK)-LDE*sin(qB-qD-qK)-LEF*sin(qB-qD-qK)))-cos(qo1+qo2)*((LDE+LEF)*cos(qG-qK)*cos(qB-qD-qK)*(LCD*cos(qB-qK)+LCI*sin(qB-qK)+LDE*cos(qB-qD-qK)-LEJ*sin(qB-qD-qK))+cos(qG-qK)*(LDE*cos(qB-qD-qK)-LEJ*sin(qB-qD-qK))*(LBH*cos(qK)+LHG*sin(qK)-LBC*cos(qB-qK)-LCD*cos(qB-qK)-LDE*cos(qB-qD-qK)-LEF*cos(qB-qD-qK))+sin(qG-qK)*((LDE+LEF)*sin(qB-qD-qK)*(LCD*cos(qB-qK)+LCI*sin(qB-qK)+LDE*cos(qB-qD-qK)-LEJ*sin(qB-qD-qK))+(LDE*cos(qB-qD-qK)-LEJ*sin(qB-qD-qK))*(LHG*cos(qK)-LBH*sin(qK)-LBC*sin(qB-qK)-LCD*sin(qB-qK)-LDE*sin(qB-qD-qK)-LEF*sin(qB-qD-qK)))))))) - 2*q_dif1*abs(((LDE+LEF)*sin(qo2)*cos(qB-qD-qG)*(LKB*sin(qK)-LBC*sin(qB-qK)-LCI*cos(qB-qK))-cos(qo1)*((LDE+LEF)*cos(qB-qD-qG)*(cos(qo1+qo2)*(LCD*cos(qB-qK)+LCI*sin(qB-qK)+LDE*cos(qB-qD-qK)-LEJ*sin(qB-qD-qK))-sin(qo1+qo2)*(LCI*cos(qB-qK)-LCD*sin(qB-qK)-LDE*sin(qB-qD-qK)-LEJ*cos(qB-qD-qK)))+(sin(qo1+qo2)*(LDE*sin(qB-qD-qK)+LEJ*cos(qB-qD-qK))+cos(qo1+qo2)*(LDE*cos(qB-qD-qK)-LEJ*sin(qB-qD-qK)))*(cos(qG-qK)*(LBH*cos(qK)+LHG*sin(qK)-LBC*cos(qB-qK)-LCD*cos(qB-qK)-LDE*cos(qB-qD-qK)-LEF*cos(qB-qD-qK))+sin(qG-qK)*(LHG*cos(qK)-LBH*sin(qK)-LBC*sin(qB-qK)-LCD*sin(qB-qK)-LDE*sin(qB-qD-qK)-LEF*sin(qB-qD-qK)))))^2*(cos(qN)+sin(qN)^2*((LDE+LEF)*cos(qo1)*sin(qo1+qo2)*cos(qB-qD-qG)*(LKB*sin(qK)-LBC*sin(qB-qK)-LCD*sin(qB-qK)-LDE*sin(qB-qD-qK)-LEJ*cos(qB-qD-qK))-(LDE+LEF)*sin(qo1)*cos(qo1+qo2)*cos(qB-qD-qG)*(LKB*sin(qK)-LBC*sin(qB-qK)-LCI*cos(qB-qK))-cos(qo1)*sin(qo1+qo2)*(LDE*sin(qB-qD-qK)+LEJ*cos(qB-qD-qK))*(cos(qG-qK)*(LBH*cos(qK)+LHG*sin(qK)-LBC*cos(qB-qK)-LCD*cos(qB-qK)-LDE*cos(qB-qD-qK)-LEF*cos(qB-qD-qK))+sin(qG-qK)*(LHG*cos(qK)-LBH*sin(qK)-LBC*sin(qB-qK)-LCD*sin(qB-qK)-LDE*sin(qB-qD-qK)-LEF*sin(qB-qD-qK)))-cos(qo1)*cos(qo1+qo2)*((LDE+LEF)*cos(qG-qK)*cos(qB-qD-qK)*(LCD*cos(qB-qK)+LCI*sin(qB-qK)+LDE*cos(qB-qD-qK)-LEJ*sin(qB-qD-qK))+cos(qG-qK)*(LDE*cos(qB-qD-qK)-LEJ*sin(qB-qD-qK))*(LBH*cos(qK)+LHG*sin(qK)-LBC*cos(qB-qK)-LCD*cos(qB-qK)-LDE*cos(qB-qD-qK)-LEF*cos(qB-qD-qK))+sin(qG-qK)*((LDE+LEF)*sin(qB-qD-qK)*(LCD*cos(qB-qK)+LCI*sin(qB-qK)+LDE*cos(qB-qD-qK)-LEJ*sin(qB-qD-qK))+(LDE*cos(qB-qD-qK)-LEJ*sin(qB-qD-qK))*(LHG*cos(qK)-LBH*sin(qK)-LBC*sin(qB-qK)-LCD*sin(qB-qK)-LDE*sin(qB-qD-qK)-LEF*sin(qB-qD-qK)))))/(cos(qN)*((LDE+LEF)*sin(qo2)*cos(qB-qD-qG)*(LKB*sin(qK)-LBC*sin(qB-qK)-LCI*cos(qB-qK))-cos(qo1)*((LDE+LEF)*cos(qB-qD-qG)*(cos(qo1+qo2)*(LCD*cos(qB-qK)+LCI*sin(qB-qK)+LDE*cos(qB-qD-qK)-LEJ*sin(qB-qD-qK))-sin(qo1+qo2)*(LCI*cos(qB-qK)-LCD*sin(qB-qK)-LDE*sin(qB-qD-qK)-LEJ*cos(qB-qD-qK)))+(sin(qo1+qo2)*(LDE*sin(qB-qD-qK)+LEJ*cos(qB-qD-qK))+cos(qo1+qo2)*(LDE*cos(qB-qD-qK)-LEJ*sin(qB-qD-qK)))*(cos(qG-qK)*(LBH*cos(qK)+LHG*sin(qK)-LBC*cos(qB-qK)-LCD*cos(qB-qK)-LDE*cos(qB-qD-qK)-LEF*cos(qB-qD-qK))+sin(qG-qK)*(LHG*cos(qK)-LBH*sin(qK)-LBC*sin(qB-qK)-LCD*sin(qB-qK)-LDE*sin(qB-qD-qK)-LEF*sin(qB-qD-qK)))))))*(LIIp*sin(qo1)+c1*cos(qo1)+((LDE+LEF)*c2*cos(qB-qD-qG)*(cos(qo1)*(LKB*cos(qK)+LBC*cos(qB-qK)-LCI*sin(qB-qK))-sin(qo1)*(LKB*sin(qK)-LBC*sin(qB-qK)-LCI*cos(qB-qK)))+(LDE+LEF)*sin(qo1+qo2)*cos(qB-qD-qG)*(LIIp*cos(qo1)+sin(qo1)*(LLM-c1))*(cos(qo1)*(LKB*cos(qK)+LBC*cos(qB-qK)-LCI*sin(qB-qK))-sin(qo1)*(LKB*sin(qK)-LBC*sin(qB-qK)-LCI*cos(qB-qK)))-(LDE+LEF)*cos(qo1+qo2)*cos(qB-qD-qG)*(LIIp*sin(qo1)-cos(qo1)*(LLM-c1))*(cos(qo1)*(LKB*cos(qK)+LBC*cos(qB-qK)-LCI*sin(qB-qK))-sin(qo1)*(LKB*sin(qK)-LBC*sin(qB-qK)-LCI*cos(qB-qK)))-(LIIp*cos(qo1)-c1*sin(qo1))*((LDE+LEF)*sin(qo2)*cos(qB-qD-qG)*(LKB*cos(qK)+LBC*cos(qB-qK)-LCI*sin(qB-qK))+sin(qo1)*((LDE+LEF)*sin(qo1+qo2)*cos(qB-qD-qG)*(LCI*cos(qB-qK)-LCD*sin(qB-qK)-LDE*sin(qB-qD-qK)-LEJ*cos(qB-qD-qK))-sin(qo1+qo2)*(LDE*sin(qB-qD-qK)+LEJ*cos(qB-qD-qK))*(cos(qG-qK)*(LBH*cos(qK)+LHG*sin(qK)-LBC*cos(qB-qK)-LCD*cos(qB-qK)-LDE*cos(qB-qD-qK)-LEF*cos(qB-qD-qK))+sin(qG-qK)*(LHG*cos(qK)-LBH*sin(qK)-LBC*sin(qB-qK)-LCD*sin(qB-qK)-LDE*sin(qB-qD-qK)-LEF*sin(qB-qD-qK)))-cos(qo1+qo2)*((LDE+LEF)*cos(qG-qK)*cos(qB-qD-qK)*(LCD*cos(qB-qK)+LCI*sin(qB-qK)+LDE*cos(qB-qD-qK)-LEJ*sin(qB-qD-qK))+cos(qG-qK)*(LDE*cos(qB-qD-qK)-LEJ*sin(qB-qD-qK))*(LBH*cos(qK)+LHG*sin(qK)-LBC*cos(qB-qK)-LCD*cos(qB-qK)-LDE*cos(qB-qD-qK)-LEF*cos(qB-qD-qK))+sin(qG-qK)*((LDE+LEF)*sin(qB-qD-qK)*(LCD*cos(qB-qK)+LCI*sin(qB-qK)+LDE*cos(qB-qD-qK)-LEJ*sin(qB-qD-qK))+(LDE*cos(qB-qD-qK)-LEJ*sin(qB-qD-qK))*(LHG*cos(qK)-LBH*sin(qK)-LBC*sin(qB-qK)-LCD*sin(qB-qK)-LDE*sin(qB-qD-qK)-LEF*sin(qB-qD-qK)))))))/((LDE+LEF)*sin(qo2)*cos(qB-qD-qG)*(LKB*sin(qK)-LBC*sin(qB-qK)-LCI*cos(qB-qK))-cos(qo1)*((LDE+LEF)*cos(qB-qD-qG)*(cos(qo1+qo2)*(LCD*cos(qB-qK)+LCI*sin(qB-qK)+LDE*cos(qB-qD-qK)-LEJ*sin(qB-qD-qK))-sin(qo1+qo2)*(LCI*cos(qB-qK)-LCD*sin(qB-qK)-LDE*sin(qB-qD-qK)-LEJ*cos(qB-qD-qK)))+(sin(qo1+qo2)*(LDE*sin(qB-qD-qK)+LEJ*cos(qB-qD-qK))+cos(qo1+qo2)*(LDE*cos(qB-qD-qK)-LEJ*sin(qB-qD-qK)))*(cos(qG-qK)*(LBH*cos(qK)+LHG*sin(qK)-LBC*cos(qB-qK)-LCD*cos(qB-qK)-LDE*cos(qB-qD-qK)-LEF*cos(qB-qD-qK))+sin(qG-qK)*(LHG*cos(qK)-LBH*sin(qK)-LBC*sin(qB-qK)-LCD*sin(qB-qK)-LDE*sin(qB-qD-qK)-LEF*sin(qB-qD-qK))))))/((LDE+LEF)*c2*cos(qB-qD-qG)*(LKB*sin(qK)+LAB*sin(qB-qK)-tan(qN)*(LKB*cos(qK)-LAB*cos(qB-qK)))*((LDE+LEF)*sin(qo1)*sin(qo2)*cos(qB-qD-qG)*(LIIp*cos(qo1)-c1*sin(qo1))*(LKB*sin(qK)-LBC*sin(qB-qK)-LCI*cos(qB-qK))-cos(qo1)*((LIIp*sin(qo1)+c1*cos(qo1))*((LDE+LEF)*sin(qo2)*cos(qB-qD-qG)*(LKB*sin(qK)-LBC*sin(qB-qK)-LCI*cos(qB-qK))-cos(qo1)*((LDE+LEF)*cos(qB-qD-qG)*(cos(qo1+qo2)*(LCD*cos(qB-qK)+LCI*sin(qB-qK)+LDE*cos(qB-qD-qK)-LEJ*sin(qB-qD-qK))-sin(qo1+qo2)*(LCI*cos(qB-qK)-LCD*sin(qB-qK)-LDE*sin(qB-qD-qK)-LEJ*cos(qB-qD-qK)))+(sin(qo1+qo2)*(LDE*sin(qB-qD-qK)+LEJ*cos(qB-qD-qK))+cos(qo1+qo2)*(LDE*cos(qB-qD-qK)-LEJ*sin(qB-qD-qK)))*(cos(qG-qK)*(LBH*cos(qK)+LHG*sin(qK)-LBC*cos(qB-qK)-LCD*cos(qB-qK)-LDE*cos(qB-qD-qK)-LEF*cos(qB-qD-qK))+sin(qG-qK)*(LHG*cos(qK)-LBH*sin(qK)-LBC*sin(qB-qK)-LCD*sin(qB-qK)-LDE*sin(qB-qD-qK)-LEF*sin(qB-qD-qK)))))-sin(qo1)*(LIIp*cos(qo1)-c1*sin(qo1))*((LDE+LEF)*sin(qo1+qo2)*cos(qB-qD-qG)*(LCI*cos(qB-qK)-LCD*sin(qB-qK)-LDE*sin(qB-qD-qK)-LEJ*cos(qB-qD-qK))-sin(qo1+qo2)*(LDE*sin(qB-qD-qK)+LEJ*cos(qB-qD-qK))*(cos(qG-qK)*(LBH*cos(qK)+LHG*sin(qK)-LBC*cos(qB-qK)-LCD*cos(qB-qK)-LDE*cos(qB-qD-qK)-LEF*cos(qB-qD-qK))+sin(qG-qK)*(LHG*cos(qK)-LBH*sin(qK)-LBC*sin(qB-qK)-LCD*sin(qB-qK)-LDE*sin(qB-qD-qK)-LEF*sin(qB-qD-qK)))-cos(qo1+qo2)*((LDE+LEF)*cos(qG-qK)*cos(qB-qD-qK)*(LCD*cos(qB-qK)+LCI*sin(qB-qK)+LDE*cos(qB-qD-qK)-LEJ*sin(qB-qD-qK))+cos(qG-qK)*(LDE*cos(qB-qD-qK)-LEJ*sin(qB-qD-qK))*(LBH*cos(qK)+LHG*sin(qK)-LBC*cos(qB-qK)-LCD*cos(qB-qK)-LDE*cos(qB-qD-qK)-LEF*cos(qB-qD-qK))+sin(qG-qK)*((LDE+LEF)*sin(qB-qD-qK)*(LCD*cos(qB-qK)+LCI*sin(qB-qK)+LDE*cos(qB-qD-qK)-LEJ*sin(qB-qD-qK))+(LDE*cos(qB-qD-qK)-LEJ*sin(qB-qD-qK))*(LHG*cos(qK)-LBH*sin(qK)-LBC*sin(qB-qK)-LCD*sin(qB-qK)-LDE*sin(qB-qD-qK)-LEF*sin(qB-qD-qK)))))))))/q_dif2 - ((LDE+LEF)*sin(qo2)*cos(qB-qD-qG)*(LKB*sin(qK)-LBC*sin(qB-qK)-LCI*cos(qB-qK))-cos(qo1)*((LDE+LEF)*cos(qB-qD-qG)*(cos(qo1+qo2)*(LCD*cos(qB-qK)+LCI*sin(qB-qK)+LDE*cos(qB-qD-qK)-LEJ*sin(qB-qD-qK))-sin(qo1+qo2)*(LCI*cos(qB-qK)-LCD*sin(qB-qK)-LDE*sin(qB-qD-qK)-LEJ*cos(qB-qD-qK)))+(sin(qo1+qo2)*(LDE*sin(qB-qD-qK)+LEJ*cos(qB-qD-qK))+cos(qo1+qo2)*(LDE*cos(qB-qD-qK)-LEJ*sin(qB-qD-qK)))*(cos(qG-qK)*(LBH*cos(qK)+LHG*sin(qK)-LBC*cos(qB-qK)-LCD*cos(qB-qK)-LDE*cos(qB-qD-qK)-LEF*cos(qB-qD-qK))+sin(qG-qK)*(LHG*cos(qK)-LBH*sin(qK)-LBC*sin(qB-qK)-LCD*sin(qB-qK)-LDE*sin(qB-qD-qK)-LEF*sin(qB-qD-qK)))))^2*(LIIp*sin(qo1)+c1*cos(qo1)+((LDE+LEF)*c2*cos(qB-qD-qG)*(cos(qo1)*(LKB*cos(qK)+LBC*cos(qB-qK)-LCI*sin(qB-qK))-sin(qo1)*(LKB*sin(qK)-LBC*sin(qB-qK)-LCI*cos(qB-qK)))+(LDE+LEF)*sin(qo1+qo2)*cos(qB-qD-qG)*(LIIp*cos(qo1)+sin(qo1)*(LLM-c1))*(cos(qo1)*(LKB*cos(qK)+LBC*cos(qB-qK)-LCI*sin(qB-qK))-sin(qo1)*(LKB*sin(qK)-LBC*sin(qB-qK)-LCI*cos(qB-qK)))-(LDE+LEF)*cos(qo1+qo2)*cos(qB-qD-qG)*(LIIp*sin(qo1)-cos(qo1)*(LLM-c1))*(cos(qo1)*(LKB*cos(qK)+LBC*cos(qB-qK)-LCI*sin(qB-qK))-sin(qo1)*(LKB*sin(qK)-LBC*sin(qB-qK)-LCI*cos(qB-qK)))-(LIIp*cos(qo1)-c1*sin(qo1))*((LDE+LEF)*sin(qo2)*cos(qB-qD-qG)*(LKB*cos(qK)+LBC*cos(qB-qK)-LCI*sin(qB-qK))+sin(qo1)*((LDE+LEF)*sin(qo1+qo2)*cos(qB-qD-qG)*(LCI*cos(qB-qK)-LCD*sin(qB-qK)-LDE*sin(qB-qD-qK)-LEJ*cos(qB-qD-qK))-sin(qo1+qo2)*(LDE*sin(qB-qD-qK)+LEJ*cos(qB-qD-qK))*(cos(qG-qK)*(LBH*cos(qK)+LHG*sin(qK)-LBC*cos(qB-qK)-LCD*cos(qB-qK)-LDE*cos(qB-qD-qK)-LEF*cos(qB-qD-qK))+sin(qG-qK)*(LHG*cos(qK)-LBH*sin(qK)-LBC*sin(qB-qK)-LCD*sin(qB-qK)-LDE*sin(qB-qD-qK)-LEF*sin(qB-qD-qK)))-cos(qo1+qo2)*((LDE+LEF)*cos(qG-qK)*cos(qB-qD-qK)*(LCD*cos(qB-qK)+LCI*sin(qB-qK)+LDE*cos(qB-qD-qK)-LEJ*sin(qB-qD-qK))+cos(qG-qK)*(LDE*cos(qB-qD-qK)-LEJ*sin(qB-qD-qK))*(LBH*cos(qK)+LHG*sin(qK)-LBC*cos(qB-qK)-LCD*cos(qB-qK)-LDE*cos(qB-qD-qK)-LEF*cos(qB-qD-qK))+sin(qG-qK)*((LDE+LEF)*sin(qB-qD-qK)*(LCD*cos(qB-qK)+LCI*sin(qB-qK)+LDE*cos(qB-qD-qK)-LEJ*sin(qB-qD-qK))+(LDE*cos(qB-qD-qK)-LEJ*sin(qB-qD-qK))*(LHG*cos(qK)-LBH*sin(qK)-LBC*sin(qB-qK)-LCD*sin(qB-qK)-LDE*sin(qB-qD-qK)-LEF*sin(qB-qD-qK)))))))/((LDE+LEF)*sin(qo2)*cos(qB-qD-qG)*(LKB*sin(qK)-LBC*sin(qB-qK)-LCI*cos(qB-qK))-cos(qo1)*((LDE+LEF)*cos(qB-qD-qG)*(cos(qo1+qo2)*(LCD*cos(qB-qK)+LCI*sin(qB-qK)+LDE*cos(qB-qD-qK)-LEJ*sin(qB-qD-qK))-sin(qo1+qo2)*(LCI*cos(qB-qK)-LCD*sin(qB-qK)-LDE*sin(qB-qD-qK)-LEJ*cos(qB-qD-qK)))+(sin(qo1+qo2)*(LDE*sin(qB-qD-qK)+LEJ*cos(qB-qD-qK))+cos(qo1+qo2)*(LDE*cos(qB-qD-qK)-LEJ*sin(qB-qD-qK)))*(cos(qG-qK)*(LBH*cos(qK)+LHG*sin(qK)-LBC*cos(qB-qK)-LCD*cos(qB-qK)-LDE*cos(qB-qD-qK)-LEF*cos(qB-qD-qK))+sin(qG-qK)*(LHG*cos(qK)-LBH*sin(qK)-LBC*sin(qB-qK)-LCD*sin(qB-qK)-LDE*sin(qB-qD-qK)-LEF*sin(qB-qD-qK))))))*(LAB*sin(qB-qK)-((LDE+LEF)*cos(qo1)*sin(qo1+qo2)*cos(qB-qD-qG)*(LKB*sin(qK)+LAB*sin(qB-qK)-tan(qN)*(LKB*cos(qK)-LAB*cos(qB-qK)))*(LCI*cos(qB-qK)-LCD*sin(qB-qK)-LDE*sin(qB-qD-qK)-LEJ*cos(qB-qD-qK))+cos(qo1)*sin(qG-qK)*(LKB*sin(qK)+LAB*sin(qB-qK)-tan(qN)*(LKB*cos(qK)-LAB*cos(qB-qK)))*(LBC*sin(qB-qK)+LCD*sin(qB-qK)+LDE*sin(qB-qD-qK)+LEF*sin(qB-qD-qK))*(sin(qo1+qo2)*(LDE*sin(qB-qD-qK)+LEJ*cos(qB-qD-qK))+cos(qo1+qo2)*(LDE*cos(qB-qD-qK)-LEJ*sin(qB-qD-qK)))+cos(qo1)*cos(qG-qK)*(LKB*sin(qK)+LAB*sin(qB-qK)-tan(qN)*(LKB*cos(qK)-LAB*cos(qB-qK)))*(LBC*cos(qB-qK)+LCD*cos(qB-qK)+LDE*cos(qB-qD-qK)+LEF*cos(qB-qD-qK))*(sin(qo1+qo2)*(LDE*sin(qB-qD-qK)+LEJ*cos(qB-qD-qK))+cos(qo1+qo2)*(LDE*cos(qB-qD-qK)-LEJ*sin(qB-qD-qK)))-(LDE+LEF)*sin(qo2)*cos(qB-qD-qG)*(LBC*sin(qB-qK)+LCI*cos(qB-qK))*(LKB*sin(qK)+LAB*sin(qB-qK)-tan(qN)*(LKB*cos(qK)-LAB*cos(qB-qK)))-(LDE+LEF)*cos(qo1)*cos(qo1+qo2)*cos(qB-qD-qG)*(LKB*sin(qK)+LAB*sin(qB-qK)-tan(qN)*(LKB*cos(qK)-LAB*cos(qB-qK)))*(LCD*cos(qB-qK)+LCI*sin(qB-qK)+LDE*cos(qB-qD-qK)-LEJ*sin(qB-qD-qK))-LAB*tan(qN)*cos(qB-qK)*((LDE+LEF)*cos(qo1)*sin(qo1+qo2)*cos(qB-qD-qG)*(LKB*sin(qK)-LBC*sin(qB-qK)-LCD*sin(qB-qK)-LDE*sin(qB-qD-qK)-LEJ*cos(qB-qD-qK))-(LDE+LEF)*sin(qo1)*cos(qo1+qo2)*cos(qB-qD-qG)*(LKB*sin(qK)-LBC*sin(qB-qK)-LCI*cos(qB-qK))-cos(qo1)*sin(qo1+qo2)*(LDE*sin(qB-qD-qK)+LEJ*cos(qB-qD-qK))*(cos(qG-qK)*(LBH*cos(qK)+LHG*sin(qK)-LBC*cos(qB-qK)-LCD*cos(qB-qK)-LDE*cos(qB-qD-qK)-LEF*cos(qB-qD-qK))+sin(qG-qK)*(LHG*cos(qK)-LBH*sin(qK)-LBC*sin(qB-qK)-LCD*sin(qB-qK)-LDE*sin(qB-qD-qK)-LEF*sin(qB-qD-qK)))-cos(qo1)*cos(qo1+qo2)*((LDE+LEF)*cos(qG-qK)*cos(qB-qD-qK)*(LCD*cos(qB-qK)+LCI*sin(qB-qK)+LDE*cos(qB-qD-qK)-LEJ*sin(qB-qD-qK))+cos(qG-qK)*(LDE*cos(qB-qD-qK)-LEJ*sin(qB-qD-qK))*(LBH*cos(qK)+LHG*sin(qK)-LBC*cos(qB-qK)-LCD*cos(qB-qK)-LDE*cos(qB-qD-qK)-LEF*cos(qB-qD-qK))+sin(qG-qK)*((LDE+LEF)*sin(qB-qD-qK)*(LCD*cos(qB-qK)+LCI*sin(qB-qK)+LDE*cos(qB-qD-qK)-LEJ*sin(qB-qD-qK))+(LDE*cos(qB-qD-qK)-LEJ*sin(qB-qD-qK))*(LHG*cos(qK)-LBH*sin(qK)-LBC*sin(qB-qK)-LCD*sin(qB-qK)-LDE*sin(qB-qD-qK)-LEF*sin(qB-qD-qK))))))/((LDE+LEF)*sin(qo2)*cos(qB-qD-qG)*(LKB*sin(qK)-LBC*sin(qB-qK)-LCI*cos(qB-qK))-cos(qo1)*((LDE+LEF)*cos(qB-qD-qG)*(cos(qo1+qo2)*(LCD*cos(qB-qK)+LCI*sin(qB-qK)+LDE*cos(qB-qD-qK)-LEJ*sin(qB-qD-qK))-sin(qo1+qo2)*(LCI*cos(qB-qK)-LCD*sin(qB-qK)-LDE*sin(qB-qD-qK)-LEJ*cos(qB-qD-qK)))+(sin(qo1+qo2)*(LDE*sin(qB-qD-qK)+LEJ*cos(qB-qD-qK))+cos(qo1+qo2)*(LDE*cos(qB-qD-qK)-LEJ*sin(qB-qD-qK)))*(cos(qG-qK)*(LBH*cos(qK)+LHG*sin(qK)-LBC*cos(qB-qK)-LCD*cos(qB-qK)-LDE*cos(qB-qD-qK)-LEF*cos(qB-qD-qK))+sin(qG-qK)*(LHG*cos(qK)-LBH*sin(qK)-LBC*sin(qB-qK)-LCD*sin(qB-qK)-LDE*sin(qB-qD-qK)-LEF*sin(qB-qD-qK))))))/((LDE+LEF)*c2*cos(qB-qD-qG)*(LKB*sin(qK)+LAB*sin(qB-qK)-tan(qN)*(LKB*cos(qK)-LAB*cos(qB-qK)))*((LDE+LEF)*sin(qo1)*sin(qo2)*cos(qB-qD-qG)*(LIIp*cos(qo1)-c1*sin(qo1))*(LKB*sin(qK)-LBC*sin(qB-qK)-LCI*cos(qB-qK))-cos(qo1)*((LIIp*sin(qo1)+c1*cos(qo1))*((LDE+LEF)*sin(qo2)*cos(qB-qD-qG)*(LKB*sin(qK)-LBC*sin(qB-qK)-LCI*cos(qB-qK))-cos(qo1)*((LDE+LEF)*cos(qB-qD-qG)*(cos(qo1+qo2)*(LCD*cos(qB-qK)+LCI*sin(qB-qK)+LDE*cos(qB-qD-qK)-LEJ*sin(qB-qD-qK))-sin(qo1+qo2)*(LCI*cos(qB-qK)-LCD*sin(qB-qK)-LDE*sin(qB-qD-qK)-LEJ*cos(qB-qD-qK)))+(sin(qo1+qo2)*(LDE*sin(qB-qD-qK)+LEJ*cos(qB-qD-qK))+cos(qo1+qo2)*(LDE*cos(qB-qD-qK)-LEJ*sin(qB-qD-qK)))*(cos(qG-qK)*(LBH*cos(qK)+LHG*sin(qK)-LBC*cos(qB-qK)-LCD*cos(qB-qK)-LDE*cos(qB-qD-qK)-LEF*cos(qB-qD-qK))+sin(qG-qK)*(LHG*cos(qK)-LBH*sin(qK)-LBC*sin(qB-qK)-LCD*sin(qB-qK)-LDE*sin(qB-qD-qK)-LEF*sin(qB-qD-qK)))))-sin(qo1)*(LIIp*cos(qo1)-c1*sin(qo1))*((LDE+LEF)*sin(qo1+qo2)*cos(qB-qD-qG)*(LCI*cos(qB-qK)-LCD*sin(qB-qK)-LDE*sin(qB-qD-qK)-LEJ*cos(qB-qD-qK))-sin(qo1+qo2)*(LDE*sin(qB-qD-qK)+LEJ*cos(qB-qD-qK))*(cos(qG-qK)*(LBH*cos(qK)+LHG*sin(qK)-LBC*cos(qB-qK)-LCD*cos(qB-qK)-LDE*cos(qB-qD-qK)-LEF*cos(qB-qD-qK))+sin(qG-qK)*(LHG*cos(qK)-LBH*sin(qK)-LBC*sin(qB-qK)-LCD*sin(qB-qK)-LDE*sin(qB-qD-qK)-LEF*sin(qB-qD-qK)))-cos(qo1+qo2)*((LDE+LEF)*cos(qG-qK)*cos(qB-qD-qK)*(LCD*cos(qB-qK)+LCI*sin(qB-qK)+LDE*cos(qB-qD-qK)-LEJ*sin(qB-qD-qK))+cos(qG-qK)*(LDE*cos(qB-qD-qK)-LEJ*sin(qB-qD-qK))*(LBH*cos(qK)+LHG*sin(qK)-LBC*cos(qB-qK)-LCD*cos(qB-qK)-LDE*cos(qB-qD-qK)-LEF*cos(qB-qD-qK))+sin(qG-qK)*((LDE+LEF)*sin(qB-qD-qK)*(LCD*cos(qB-qK)+LCI*sin(qB-qK)+LDE*cos(qB-qD-qK)-LEJ*sin(qB-qD-qK))+(LDE*cos(qB-qD-qK)-LEJ*sin(qB-qD-qK))*(LHG*cos(qK)-LBH*sin(qK)-LBC*sin(qB-qK)-LCD*sin(qB-qK)-LDE*sin(qB-qD-qK)-LEF*sin(qB-qD-qK)))))))))/2;

if J22_c == 0 || isnan(J22_c) || isinf(J22_c)
    J22 = single(J22_old);
else
    J22 = single(-abs(J22_c));
end
% 
J22_ol = single(J22);



JTcomp = [J11; J12; J21; J22];


q_next = single(sensor);
